simulink model "Quadcopter_NMPC_2"  (R2023a)
settings: Solver=ode4  StartTime=0.0  StopTime=20  FixedStep=0.001  RelTol=1e-3
libraries: mpclib x1
settings Model: Creator=Hameed  LastModifiedBy=Hameed
settings DebuggingCC: UnconnectedInputMsg=warning  UnconnectedOutputMsg=warning  UnconnectedLineMsg=warning
settings ModelReferenceCC: EnableRefExpFcnMdlSchedulingChecks=on
settings RTWCC: DLArmComputeVersion=19.05

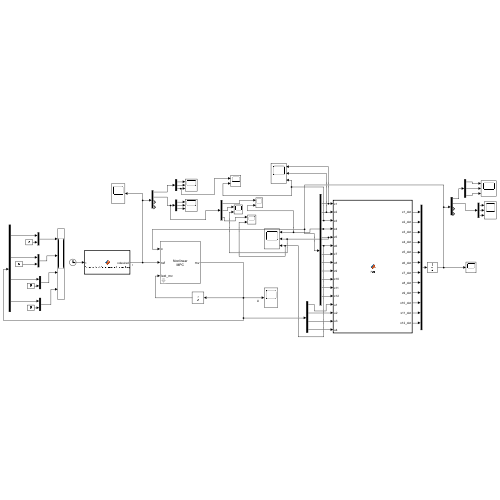
[thumbnail: Simulink's stored preview of the top-level diagram]
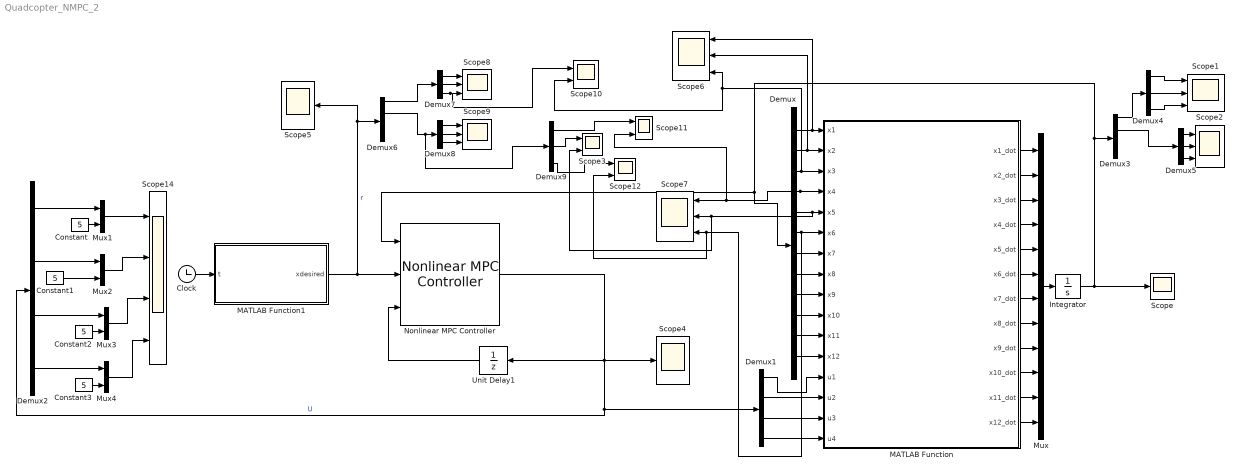
== system Quadcopter_NMPC_2 ==
  Clock : Clock
  Constant{,1..3} (4 alike) : Constant  Value=5
  Demux : Demux  Outputs=12
  Demux{1..3,6} (4 alike) : Demux
  Demux{4..5,7..9} (5 alike) : Demux  Outputs=3
  Integrator : Integrator  InitialCondition=[0;0;0.1;pi/15;0;0;0;0;0;0;0;0]
  MATLAB Function : MATLAB Function  TreatAsAtomicUnit=on
  MATLAB Function1 : MATLAB Function  TreatAsAtomicUnit=on
  Mux : Mux  Inputs=12
  Mux{1..4} (4 alike) : Mux  Inputs=2
  Nonlinear MPC Controller : mpclib/Nonlinear MPC Controller  SCDEnableBlockLinearizationSpecification=on  nlmpcobj=nlobj11  UseObjectTs=on  UseMEX=off  md_enabled=off  mvtarget_enabled=off  param_enabled=off  cost_enabled=off  mvseq_enabled=off  stateseq_enabled=off  ovseq_enabled=off  slack_enabled=off  status_enabled=off  ov_min=off  ov_max=off  mv_min=off  mv_max=off  mvrate_min=off  mvrate_max=off  state_min=off  state_max=off  ov_weight=off  mv_weight=off  mvrate_weight=off  ecr_weight=off  nlp_initialize=off
  Scope : Scope
  Scope{1..2,6..9} (6 alike) : Scope  NumInputPorts=3
  Scope{3,10..12} (4 alike) : Scope  NumInputPorts=2
  Scope14 : Scope  NumInputPorts=4
  Scope4 : Scope
  Scope5 : Scope
  Unit Delay1 : UnitDelay  InitialCondition=[0;0;0;0]  SampleTime=0.1  HasFrameUpgradeWarning=on
  wires:
  MATLAB Function/7(x7_dot) -> Mux/7
  MATLAB Function/8(x8_dot) -> Mux/8
  MATLAB Function/5(x5_dot) -> Mux/5
  MATLAB Function/2(x2_dot) -> Mux/2
  MATLAB Function/9(x9_dot) -> Mux/9
  MATLAB Function/4(x4_dot) -> Mux/4
  Nonlinear MPC Controller/1 -> Demux2/1, Demux1/1, Unit Delay1/1, Scope4/1  "U"
  Demux/5 -> MATLAB Function/5(x5), Scope3/2, Scope7/2
  Demux/9 -> MATLAB Function/9(x9)
  Demux/11 -> MATLAB Function/11(x11)
  MATLAB Function/6(x6_dot) -> Mux/6
  Integrator/1 -> Scope/1, Demux3/1, Demux/1, Nonlinear MPC Controller/1
  Mux/1 -> Integrator/1
  Demux/3 -> MATLAB Function/3(x3), Scope10/2, Scope6/3
  Demux/6 -> MATLAB Function/6(x6), Scope12/2, Scope7/3
  Demux/2 -> MATLAB Function/2(x2), Scope6/2
  Demux/10 -> MATLAB Function/10(x10)
  Demux/12 -> MATLAB Function/12(x12)
  Demux/4 -> MATLAB Function/4(x4), Scope11/2, Scope7/1
  Demux/7 -> MATLAB Function/7(x7)
  MATLAB Function/12(x12_dot) -> Mux/12
  Demux/1 -> MATLAB Function/1(x1), Scope6/1
  MATLAB Function/3(x3_dot) -> Mux/3
  MATLAB Function/1(x1_dot) -> Mux/1
  Demux1/3 -> MATLAB Function/15(u3)
  Demux1/4 -> MATLAB Function/16(u4)
  Demux1/2 -> MATLAB Function/14(u2)
  MATLAB Function1/1(xdesired) -> Nonlinear MPC Controller/2, Scope5/1, Demux6/1  "r"
  Demux/8 -> MATLAB Function/8(x8)
  MATLAB Function/11(x11_dot) -> Mux/11
  MATLAB Function/10(x10_dot) -> Mux/10
  Demux1/1 -> MATLAB Function/13(u1)
  Clock/1 -> MATLAB Function1/1(t)
  Unit Delay1/1 -> Nonlinear MPC Controller/3
  Demux2/1 -> Mux1/1
  Demux2/2 -> Mux2/1
  Demux2/3 -> Mux3/1
  Demux3/1 -> Demux4/1
  Demux3/2 -> Demux5/1
  Demux4/2 -> Scope1/2
  Demux4/1 -> Scope1/1
  Demux4/3 -> Scope1/3
  Demux5/3 -> Scope2/3
  Demux5/1 -> Scope2/1
  Demux5/2 -> Scope2/2
  Demux7/1 -> Scope8/1
  Demux7/2 -> Scope8/2
  Demux6/1 -> Demux7/1
  Demux8/1 -> Scope9/1
  Demux8/3 -> Scope9/3
  Demux8/2 -> Scope9/2
  Demux7/3 -> Scope10/1, Scope8/3
  Demux6/2 -> Demux9/1, Demux8/1
  Demux9/1 -> Scope11/1
  Demux9/2 -> Scope3/1
  Demux9/3 -> Scope12/1
  Demux2/4 -> Mux4/1
  Constant/1 -> Mux1/2
  Constant1/1 -> Mux2/2
  Constant2/1 -> Mux3/2
  Constant3/1 -> Mux4/2
  Mux2/1 -> Scope14/2
  Mux1/1 -> Scope14/1
  Mux4/1 -> Scope14/4
  Mux3/1 -> Scope14/3

== matlab function Quadcopter_NMPC_2/MATLAB Function1 ==
  data: t input; xdesired output
function xdesired   = QuadrotorReferenceTrajectory( t )
% This function generates reference signal for nonlinear MPC controller
% used in the quadrotor path following example.

% Copyright 2019 The MathWorks, Inc.

%#codegen
x =6*sin(t/3);
y = -6*sin(t/3).*cos(t/3);
z = 6*cos(t/3);
%z = 10+zeros(1,length(t));
phi = zeros(1,length(t));
theta = zeros(1,length(t));
psi = zeros(1,length(t));
% phi = pi/6*sin(t/3);
% theta = -pi/3*sin(t/3).*cos(t/3);
% psi = pi*ones(1,length(t));
xdot = zeros(1,length(t));
ydot = zeros(1,length(t));
zdot = zeros(1,length(t));
phidot = zeros(1,length(t));
thetadot = zeros(1,length(t));
psidot = zeros(1,length(t));

xdesired = [x;y;z;phi;theta;psi;xdot;ydot;zdot;phidot;thetadot;psidot]';
end

== matlab function Quadcopter_NMPC_2/MATLAB Function ==
  data: x1 input; x1_dot output; x2 input; x3 input; x4 input; x5 input; x6 input; x7 input; x8 input; x9 input; x10 input; x11 input; x12 input; u1 input; u2 input; u3 input; u4 input; x2_dot output; x3_dot output; x4_dot output; x5_dot output; x6_dot output; x7_dot output; x8_dot output; x9_dot output; x10_dot output; x11_dot output; x12_dot output
function [x1_dot,x2_dot,x3_dot,x4_dot,x5_dot,x6_dot,x7_dot,x8_dot,x9_dot,x10_dot,x11_dot,x12_dot]= fcn(x1,x2,x3,x4,x5,x6,x7,x8,x9,x10,x11,x12,u1,u2,u3,u4)
% x=x1;
% y=x2,
% z=x3
% phi=x4;
% theta=x5;
% sai=x6;
% x_dot=x7;
% y_dot=x8,
% z_dot=x9
% phi_dot=x10;
% theta_dot=x11;
% sai_dot=x12;

Ixx= 1.2; 
Iyy= 1.2;
Izz= 2.3;
k= 1;
l= 0.25;
m= 2;
b= 0.2;
g= 9.81;

% Ixx= 4.856e-3; 
% Iyy= 4.856e-3;
% Izz= 8.8e-3;
% k= 2.98e-6;
% l= 0.225;
% m= 0.468;
% b= 1.14e-7;
% g= 9.81;

T = k*(u1+u2+u3+u4);
x789= -g*[0;0;1]+(T/m)*[sin(x6)*sin(x5)*sin(x4)+sin(x6)*sin(x4);cos(x6)*cos(x5)*cos(x4)-cos(x6)*cos(x4);cos(x5)*cos(x4)];

tB= [l*k*(-u2 + u4);l*k*(-u1 + u3);b*(-u1+u2-u3+u4)];


C11=0;
C12=(Iyy-Izz)*(x7*cos(x4)*sin(x4)+x12*sin(x4)^2*cos(x5))+(Izz-Iyy)*x12*cos(x4)^2*cos(x5)-Ixx*x12*cos(x5);
C13=(Izz-Iyy)*(x12*cos(x4)*sin(x4)*cos(x5)^2);
C21=(Izz-Iyy)*(x7*cos(x4)*sin(x4)+x12*sin(x4)*cos(x5))+(Iyy-Izz)*x12*cos(x4)^2*cos(x5)-Ixx*x12*cos(x5);
C22=(Izz-Iyy)*x10*cos(x4)*sin(x4);
C23= -Ixx*x12*sin(x5)*cos(x5)+Iyy*x12*sin(x4)^2*sin(x5)*cos(x5)+ Izz*x12*cos(x4)^2*sin(x5)*cos(x5);
C31=(Iyy-Izz)*(x12*cos(x5)^2*sin(x4)*cos(x4))-Ixx*x11*cos(x5);
C32= (Izz-Iyy)*(x11*cos(x4)*sin(x4)*sin(x5)+x10*sin(x4)^2*cos(x5))+(Iyy-Izz)*x10*cos(x4)^2*cos(x5)+Ixx*x12*cos(x5)*cos(x5)-Iyy*x12*sin(x10)^2*sin(x5)*cos(x5)-Izz*x12*cos(x10)^2*sin(x5)*cos(x5);
C33=(Iyy-Izz)*x10*cos(x4)*sin(x4)*cos(x5)^2-Iyy*x11*sin(x4)^2*cos(x5)*sin(x5)-Izz*x11*cos(x4)^2*cos(x5)*sin(x5)+Ixx*x11*cos(x5)*sin(x5);
Cnndot=[C11 C12 C13;C21 C22 C23;C31 C32 C33];

%ndot=[x10_dot;x11_dot;x12_dot];
ndot=[x10;x11;x12];


W = [1, 0, -sin(x5);
    0, cos(x4), cos(x5)*sin(x4);
    0, -sin(x4), cos(x5)*cos(x4)];
I = [Ixx,0,0;0,Iyy,0;0,0,Izz];
J = W.'*I*W;
Jinv=inv(J)
x101112= Jinv*(tB-Cnndot*ndot);

x1_dot=x7;
x2_dot=x8;
x3_dot=x9;
x4_dot=x10;
x5_dot=x11;
x6_dot=x12;
x7_dot=x789(1);
x8_dot=x789(2);
x9_dot=x789(3);
x10_dot=x101112(1);
x11_dot=x101112(2);
x12_dot=x101112(3);


%y=u;
